simulink model "UncontrolledRectifier"  (R2023a)
settings: Solver=VariableStepAuto  StartTime=0.0  StopTime=10.0  RelTol=1e-3
libraries: spsDiodeLib x4, spsSeriesRLCBranchLib x3, spsVoltageMeasurementLib x2, spsACVoltageSourceLib x1, spsCurrentMeasurementLib x1, sps_lib x1
settings Model: Creator=Siddesh  LastModifiedBy=Siddesh

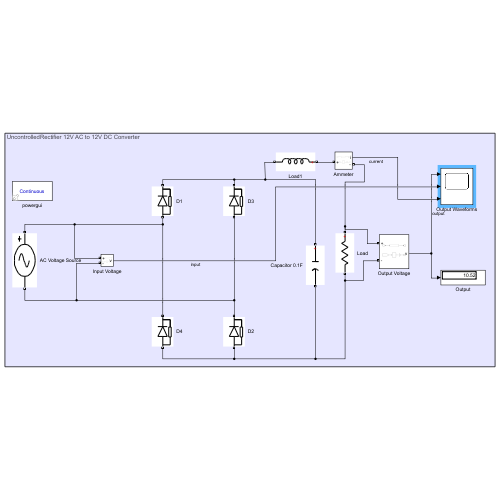
[thumbnail: Simulink's stored preview of the top-level diagram]
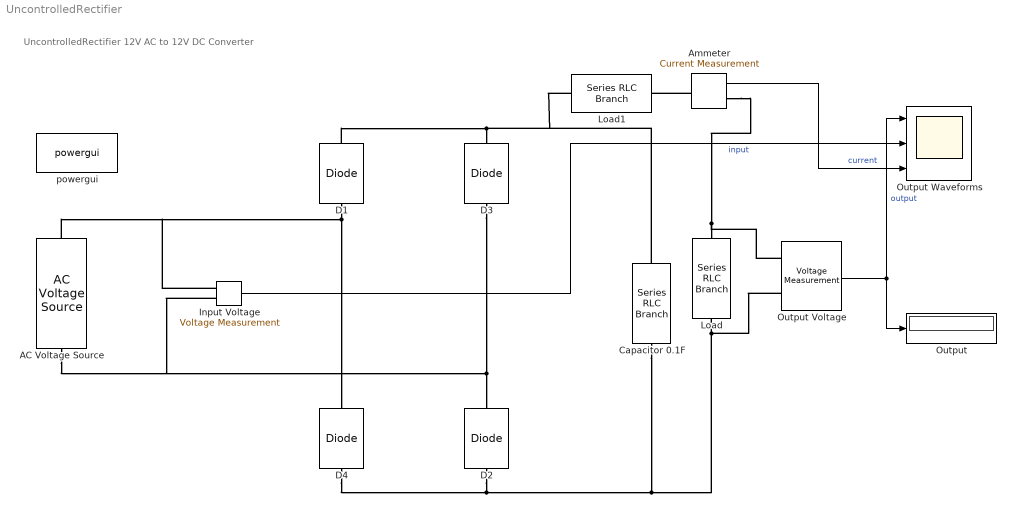
== system UncontrolledRectifier ==
  note: UncontrolledRectifier 12V AC to 12V DC Converter
  "AC Voltage Source " : spsACVoltageSourceLib/AC Voltage Source  Amplitude=12  Phase=0  Frequency=50  SampleTime=0  Measurements=None  BusType=swing  Pref=10e3  Qref=0  Qmin=-inf  Qmax=+inf
  Ammeter : spsCurrentMeasurementLib/Current Measurement  PhasorSimulation=off  OutputType=Complex  PSBequivalent=0
  Capacitor 0.1F : spsSeriesRLCBranchLib/Series RLC Branch  LConnTagsString=__new0  RConnTagsString=__new0  BranchType=C  Resistance=1  Inductance=1e-3  SetiL0=off  InitialCurrent=0  Capacitance=100000e-6  Setx0=off  InitialVoltage=0  Measurements=None
  D{1..4} (4 alike) : spsDiodeLib/Diode  Ron=0.0001  Lon=0  Vf=0.7  IC=0  UseSnubber=0  Rs=500  Cs=250e-9  Measurements=off
  Input Voltage : spsVoltageMeasurementLib/Voltage Measurement  PhasorSimulation=off  OutputType=Complex  PSBequivalent=0
  Load : spsSeriesRLCBranchLib/Series RLC Branch  LConnTagsString=__new0  RConnTagsString=__new0  BranchType=R  Resistance=12  Inductance=1e-3  SetiL0=off  InitialCurrent=0  Capacitance=1e-6  Setx0=off  InitialVoltage=0  Measurements=None
  Load1 : spsSeriesRLCBranchLib/Series RLC Branch  LConnTagsString=__new0  RConnTagsString=__new0  BranchType=L  Resistance=12  Inductance=1500e-3  SetiL0=off  InitialCurrent=0  Capacitance=1e-6  Setx0=off  InitialVoltage=0  Measurements=None
  Output : Display
  Output Voltage : spsVoltageMeasurementLib/Voltage Measurement  PhasorSimulation=off  OutputType=Complex  PSBequivalent=0
  Output Waveforms : Scope  NumInputPorts=3
  powergui : sps_lib/powergui  Priority=1  SimulationMode=Continuous  SampleTime=50e-6  frequency=60  Iterations=50  frequencyindice=50  Pbase=100e6  ErrMax=1e-4  UnitsV=kV  UnitsW=MW  buscounter=0  FunctionMessages=off  echomessages=off  EnableUseOfTLC=off  CurrentSourceSwitches=off  DisableSnubberDevices=off  DisableRonSwitches=off  DisableVfSwitches=off  DisplayEquations=off  AutomaticDiscreteSolvers=off  SolverType=Tustin/Backward Euler (TBE)  Interpol=off  ExternalGateDelay=off  methode=off  Ts=100  x0status=blocks  SPID=on  SwTol=0  HookPort=off  NonlinearTolerance=1e-4  nMaxIteration=100  ContinueOnMaxIteration=off  RestoreLinks=warning  ResistiveCurrentMeasurement=off  Frange=[0:2:500]  Ylog=off  Xlog=on  ShowGrid=off  save=off  variable=ZData  structure=0  ZoomFFT=off  StartTime=0.0  cycles=1  DisplayStyle=1  fundamental=60  FreqAxis=off  MaxFrequency=1000  frequencyindicesteady=1  RmsSteady=1  display=off
  wires:
  Output Voltage/1 -> Output/1, Output Waveforms/1  "output"
  Input Voltage/1 -> Output Waveforms/2  "input"
  Ammeter/1 -> Output Waveforms/3  "current"
  connections:
  D1/LConn1 -- Input Voltage/LConn1 -- "AC Voltage Source "/RConn1 -- D4/RConn1
  D3/LConn1 -- Input Voltage/LConn2 -- "AC Voltage Source "/LConn1 -- D2/RConn1
  D3/RConn1 -- Load1/RConn1 -- Capacitor 0.1F/LConn1 -- D1/RConn1
  D2/LConn1 -- D4/LConn1 -- Output Voltage/LConn2 -- Load/RConn1 -- Capacitor 0.1F/RConn1
  Output Voltage/LConn1 -- Ammeter/RConn1 -- Load/LConn1
  Ammeter/LConn1 -- Load1/LConn1
